simulink model "ModeAdjust"  (R2018b)
settings: Solver=FixedStepDiscrete  StartTime=0.0  StopTime=inf  FixedStep=0.01  RelTol=1e-3
undefined symbols (not defined in the file or in its folder): IfKeSMSbSeatMovBkRclnEnable_Val, IfKeSMSbSeatMovFrwdBkwdEnable_Val, IfKeSMSbSeatMovFtrstEnable_Val, IfKeSMSbSeatMovHdrstFrwdBkwdEnable_Val, IfKeSMSbSeatMovHdUpwdDnwdEnable_Val, IfKeSMSbSeatMovLgrstEnable_Val, IfKeSMSbSeatMovLtwdRtwdEnable_Val, IfVeSMSeStNumConfig, KeSMSbArmscreenMovEnable_Val, KeSMSbSeatMovLgrstExpdEnable_Val, KeSMSuFirstRwStBackPosDelta_Val, KeSMSuFirstRwStBackPosTolr_Val, KeSMSuFirstRwStCushFrntPosDelta_Val, KeSMSuFirstRwStCushFrntPosTolr_Val, KeSMSuFirstRwStCushRePosDelta_Val, KeSMSuFirstRwStCushRePosTolr_Val, KeSMSuFirstRwStFootrestPosDelta_Val, KeSMSuFirstRwStFootrestPosTolr_Val, KeSMSuFirstRwStFwdBkwdPosDelta_Val, KeSMSuFirstRwStFwdBkwdPosTolr_Val, KeSMSuMdMotFinshdTm_Val, KeSMSuMdRetryTm1_Val, KeSMSuModeReqDurgTm_Val, KeSMSuSecRwStArmTochPosDelta_Val, KeSMSuSecRwStArmTochPosTolr_Val, KeSMSuSecRwStBackPosDelta_Val, KeSMSuSecRwStBackPosTolr_Val, KeSMSuSecRwStFtrstUpwdDnwdPosDelta_Val, KeSMSuSecRwStFtrstUpwdDnwdPosTolr_Val, KeSMSuSecRwStFwdBkwdPosDelta_Val, KeSMSuSecRwStFwdBkwdPosTolr_Val, KeSMSuSecRwStHeadrestFwdBkwdPosDelta_Val, KeSMSuSecRwStHeadrestFwdBkwdPosTolr_Val, KeSMSuSecRwStHeadrestUpwdDwnwdPosDelta_Val, KeSMSuSecRwStHeadrestUpwdDwnwdPosTolr_Val, KeSMSuSecRwStLegrestInOutPosDelta_Val, KeSMSuSecRwStLegrestInOutPosTolr_Val, KeSMSuSecRwStLegrestUpwdDwnwdPosDelta_Val, KeSMSuSecRwStLegrestUpwdDwnwdPosTolr_Val, KeSMSuSecRwStLwdRwdPosDelta_Val, KeSMSuSecRwStLwdRwdPosTolr_Val, KeSMSuSecRwStVIPFtrstRefAngle_Val, KeSMSuThirdRwStFwdBkwdPosDelta_Val, KeSMSuThirdRwStFwdBkwdPosTolr_Val, KeSMSuThrdRwCushFoldPosDelta_Val, KeSMSuThrdRwCushFoldPosTolr_Val, KeSMSuThrdRwStBackPosDelta_Val, KeSMSuThrdRwStBackPosTolr_Val, KeSMSw4SLegrstCloseMdSecRwLtStFtrstUpwdDnwdPos_Val, KeSMSw4SLegrstCloseMdSecRwLtStFtrstUpwdDnwdPosMax_Val, KeSMSw4SLegrstCloseMdSecRwLtStFtrstUpwdDnwdPosMin_Val, KeSMSw4SLegrstCloseMdSecRwLtStLgrstOtwdInwdPos_Val, KeSMSw4SLegrstCloseMdSecRwLtStLgrstOtwdInwdPosMax_Val, KeSMSw4SLegrstCloseMdSecRwLtStLgrstOtwdInwdPosMin_Val, KeSMSw4SLegrstCloseMdSecRwLtStLgrstUpwdDnwdPos_Val, KeSMSw4SLegrstCloseMdSecRwLtStLgrstUpwdDnwdPosMax_Val, KeSMSw4SLegrstCloseMdSecRwLtStLgrstUpwdDnwdPosMin_Val, KeSMSw4SLegrstCloseMdSecRwRtStFtrstUpwdDnwdPos_Val, KeSMSw4SLegrstCloseMdSecRwRtStFtrstUpwdDnwdPosMax_Val, KeSMSw4SLegrstCloseMdSecRwRtStFtrstUpwdDnwdPosMin_Val ... (+1138)
libraries: Lib x401
(part 23 of 35)

== system ModeAdjust/ModeAdjustRunnable_sys/ModeAdjust/VIPR/R2Rt ==
  note: %1锁，2未锁
  Mode_Trig : Inport
  Step1En : Inport  Port=2
  Step2En : Inport  Port=3
  Step3En : Inport  Port=4
  SecRwRtStPoss : Inport  Port=5
  SecRwRtStPossV : Inport  Port=6
  SecRwRtStChldLkRsp_L : Inport  Port=7
  ModeStCalib_2R : Inport  Port=8
  StConfig : Inport  Port=9
  isSeatOccupied : Inport  Port=10
  Bus Creator : BusCreator  Inputs=9  OutDataTypeStr=Bus: SecRwRtSeatPos
  Bus Selector : BusSelector  OutputSignals=IfVeSMSuSecRwRtStBkReclnUpwdDnwdPos_Val_read,IfVeSMSuSecRwRtStFrwdBkwdPos_Val_read,IfVeSMSuSecRwRtStHPassStUpwdDnwdPos_Val_read,IfVeSMSuSecRwRtStLgrstUpwdDnwdPos_Val_read,IfVeSMSuSecRwRtStLtwdRtwdPos_Val_read,SecRwRtStArmScrnPos_Val_read
  Bus Selector1 : BusSelector  OutputSignals=IfVeSMSuSecRwRtStBkReclnUpwdDnwdPosV_Val_read,IfVeSMSuSecRwRtStFrwdBkwdPosV_Val_read,IfVeSMSuSecRwRtStHPassStUpwdDnwdPosV_Val_read,IfVeSMSuSecRwRtStLgrstUpwdDnwdPosV_Val_read,IfVeSMSuSecRwRtStLtwdRtwdPosV_Val_read,SecRwRtStArmScrnPosV_Val_read
  Bus Selector2 : BusSelector  OutputSignals=ArmScrnPos,ArmScrnPosMax,ArmScrnPosMin,BkReclnUpwdDnwdPos,BkReclnUpwdDnwdPosMax,BkReclnUpwdDnwdPosMin,FrwdBkwdPos,FrwdBkwdPosMax,FrwdBkwdPosMin,HdrstUpwdPos,HdrstUpwdPosMax,HdrstUpwdPosMin,LgrstUpwdPos,LgrstUpwdPosMax,LgrstUpwdPosMin,LtwdRtwdPos,LtwdRtwdPosMax,LtwdRtwdPosMin
  Bus Selector3 : BusSelector  OutputSignals=VIPSecRwRtSt
  Bus Selector4 : BusSelector  OutputSignals=BkReclnUpwdDnwdMovConfig,ArmTouchMovConfig,FrwdBkwdMovConfig,LgrstUpwdMovConfig,LtwdRtwdMovConfig
  Constant : Constant  Value=2  OutDataTypeStr=uint8
  Constant1 : Constant  Value=0  OutDataTypeStr=uint8
  Delay1 : Delay  DelayLength=1
  Delay2 : Delay  DelayLength=1
  Delay4 : Delay  DelayLength=1
  Logical Operator{1..3,5..6,10} (6 alike) : Logic  AllPortsSameDT=off  OutDataTypeStr=boolean
  Logical Operator{4,11..12,16} (4 alike) : Logic  Operator=OR  AllPortsSameDT=off  OutDataTypeStr=boolean
  Logical Operator15 : Logic  Inputs=3  AllPortsSameDT=off  OutDataTypeStr=boolean
  PA_KeSMSuMdMotFinshdTm_Val : Constant  Value=KeSMSuMdMotFinshdTm_Val
  PA_KeSMSuMdRetryTm1_Val : Constant  Value=KeSMSuMdRetryTm1_Val
  PA_KeSMSuModeReqDurgTm_Val : Constant  Value=KeSMSuModeReqDurgTm_Val
  PA_KeSMSuSecRwStArmTochPosDelta_Val : Constant  Value=KeSMSuSecRwStArmTochPosDelta_Val
  PA_KeSMSuSecRwStBackPosDelta_Val : Constant  Value=KeSMSuSecRwStBackPosDelta_Val
  PA_KeSMSuSecRwStFwdBkwdPosDelta_Val : Constant  Value=KeSMSuSecRwStFwdBkwdPosDelta_Val
  PA_KeSMSuSecRwStLegrestUpwdDwnwdPosDelta_Val : Constant  Value=KeSMSuSecRwStLegrestUpwdDwnwdPosDelta_Val
  PA_KeSMSuSecRwStLwdRwdPosDelta_Val : Constant  Value=KeSMSuSecRwStLwdRwdPosDelta_Val
  PA_KeSMSwDltTrgtPos_Val{1,3,6,10,12,17,19..22} (10 alike) : Constant  Value=KeSMSwPosInvalidVal_Val
  PA_KeSMSwDltTrgtPos_Val18 : Constant  OutDataTypeStr=boolean
  PA_KeSMSwDltTrgtPos_Val2 : Constant  Value=SeatChldLkSt.ChldLkSt_Unlock
  PA_KeSMSwDltTrgtPos_Val4 : Constant  Value=0  OutDataTypeStr=boolean
  PA_KeSMSwDltTrgtPos_Val5 : Constant  Value=0  OutDataTypeStr=boolean
  PA_KeSMSwDltTrgtPos_Val8 : Constant  Value=0  OutDataTypeStr=boolean
  R2LtSt_BkReclnUpwdDnwd_Lt_Step1 : Subsystem
  R2RtSt_LgrstUpwd_Step3 : Lib/CommonUsed  SystemSampleTime=-1
  R2Rt_LtwdRtwd_Step2 : Lib/CommonUsed  SystemSampleTime=-1
  Relational Operator : RelationalOperator  Operator=~=  OutDataTypeStr=boolean  RndMeth=Simplest
  Relational Operator2 : RelationalOperator  Operator=~=  OutDataTypeStr=boolean  RndMeth=Simplest
  SecRwRtStFrwdBkwd_Step2 : Lib/CommonUsed  SystemSampleTime=-1
  Switch : Switch  Criteria=u2 ~= 0
  Unit Delay : UnitDelay  SampleTime=-1
  R2RtSt_Step1_ini : Outport
  ini_ReclnOverUp : Outport  Port=2
  ini_ReclnOverDwn : Outport  Port=3
  R2RtSt_Step2_ini : Outport  Port=4
  R2Rt_Step1_done : Outport  Port=5
  R2Rt_Step2_done : Outport  Port=6
  R2Rt_TrgtPoss : Outport  Port=7  VectorParamsAs1DForOutWhenUnconnected=on
  R2RtSt_Step3_ini : Outport  Port=8
  R2Rt_Step3_done : Outport  Port=9
  IfVeSMSbSecRwRtStRclCmdSrv_Val_writeRaw : Outport  Port=10
  R2Rt_All_done : Outport  Port=11
  R2Rt_SpdCtrl : Outport  Port=12  VectorParamsAs1DForOutWhenUnconnected=on
  wires:
  PA_KeSMSwDltTrgtPos_Val8/1 -> R2Rt_LtwdRtwd_Step2/13
  PA_KeSMSwDltTrgtPos_Val5/1 -> SecRwRtStFrwdBkwd_Step2/13
  PA_KeSMSwDltTrgtPos_Val4/1 -> R2RtSt_LgrstUpwd_Step3/13
  ModeStCalib_2R/1 -> Bus Selector3/1
  Bus Selector2/6 -> [K_BkReclnUpwdDnwdPosMin]  "<BkReclnUpwdDnwdPosMin>"
  Bus Selector2/2 -> [K_ArmScrnPosMax]  "<ArmScrnPosMax>"
  Bus Selector2/3 -> [K_ArmScrnPosMin]  "<ArmScrnPosMin>"
  Bus Selector2/7 -> [K_FrwdBkwdPos]  "<FrwdBkwdPos>"
  Bus Selector3/1 -> Bus Selector2/1  "<VIPSecRwRtSt>"
  Bus Selector2/8 -> [K_FrwdBkwdPosMax]  "<FrwdBkwdPosMax>"
  Bus Selector2/5 -> [K_BkReclnUpwdDnwdPosMax]  "<BkReclnUpwdDnwdPosMax>"
  Bus Selector2/9 -> [K_FrwdBkwdPosMin]  "<FrwdBkwdPosMin>"
  Bus Selector2/4 -> [K_BkReclnUpwdDnwdPos]  "<BkReclnUpwdDnwdPos>"
  Bus Selector2/10 -> [K_HdrstUpwdPos]  "<HdrstUpwdPos>"
  Bus Selector2/14 -> [K_LgrstUpwdPosMax]  "<LgrstUpwdPosMax>"
  Bus Selector2/11 -> [K_HdrstUpwdPosMax]  "<HdrstUpwdPosMax>"
  Bus Selector2/13 -> [K_LgrstUpwdPos]  "<LgrstUpwdPos>"
  Bus Selector2/12 -> [K_HdrstUpwdPosMin]  "<HdrstUpwdPosMin>"
  Bus Selector2/17 -> [K_LtwdRtwdPosMax]  "<LtwdRtwdPosMax>"
  Bus Selector2/15 -> [K_LgrstUpwdPosMin]  "<LgrstUpwdPosMin>"
  Bus Selector2/16 -> [K_LtwdRtwdPos]  "<LtwdRtwdPos>"
  Bus Selector2/18 -> [K_LtwdRtwdPosMin]  "<LtwdRtwdPosMin>"
  Bus Selector2/1 -> [K_ArmScrnPos]  "<ArmScrnPos>"
  Bus Selector1/6 -> [SecRwRtStArmScrnPosV]  "<SecRwRtStArmScrnPosV_Val_read>"
  Bus Selector/6 -> [SecRwRtStArmScrnPos]  "<SecRwRtStArmScrnPos_Val_read>"
  [KeSMSuMdMotFinshdTm_Val] -> SecRwRtStFrwdBkwd_Step2/12
  [KeSMSuMdMotFinshdTm_Val] -> R2Rt_LtwdRtwd_Step2/12
  [KeSMSuMdMotFinshdTm_Val] -> R2RtSt_LgrstUpwd_Step3/12
  [KeSMSuMdMotFinshdTm_Val] -> R2LtSt_BkReclnUpwdDnwd_Lt_Step1/13(CheckFinishTm)
  PA_KeSMSuSecRwStArmTochPosDelta_Val/1 -> [KeSMSuSecRwStArmTochPosDelta_Val]
  PA_KeSMSuMdMotFinshdTm_Val/1 -> [KeSMSuMdMotFinshdTm_Val]
  PA_KeSMSuSecRwStBackPosDelta_Val/1 -> [KeSMSuSecRwStBackPosDelta_Val]
  PA_KeSMSuSecRwStLwdRwdPosDelta_Val/1 -> [KeSMSuSecRwStLwdRwdPosDelta_Val]
  PA_KeSMSuSecRwStLegrestUpwdDwnwdPosDelta_Val/1 -> [KeSMSuSecRwStLegrestUpwdDwnwdPosDelta_Val]
  PA_KeSMSuSecRwStFwdBkwdPosDelta_Val/1 -> [KeSMSuSecRwStFwdBkwdPosDelta_Val]
  PA_KeSMSwDltTrgtPos_Val1/1 -> Bus Creator/9  "SecRwRtStArmScrnTrgtPos"
  [Step3_1_done] -> Logical Operator10/1
  R2LtSt_BkReclnUpwdDnwd_Lt_Step1/7(Stg_done3) -> [Step3_1_done]
  R2LtSt_BkReclnUpwdDnwd_Lt_Step1/5(TarPos) -> [R2RtSt_BkReclnUpwdDnwd_TarPos]
  [Step3En] -> R2LtSt_BkReclnUpwdDnwd_Lt_Step1/3(Ena3)
  [Step1En] -> R2LtSt_BkReclnUpwdDnwd_Lt_Step1/2(Ena1)
  PA_KeSMSuModeReqDurgTm_Val/1 -> [Tick]
  [SecRwRtStLtwdRtwdPosV] -> R2Rt_LtwdRtwd_Step2/8
  [K_LgrstUpwdPos] -> R2RtSt_LgrstUpwd_Step3/6
  [K_LgrstUpwdPosMax] -> R2RtSt_LgrstUpwd_Step3/5
  [K_LgrstUpwdPosMin] -> R2RtSt_LgrstUpwd_Step3/4
  [Step3done] -> Logical Operator15/3
  [Step2done] -> Logical Operator15/2
  [Step1done_1] -> Logical Operator15/1
  [R2Rt_Step3_2_ini] -> Logical Operator16/1
  Unit Delay/1 -> Logical Operator16/2
  Logical Operator15/1 -> R2Rt_All_done/1
  Logical Operator12/1 -> R2Rt_Step3_done/1, [Step3done]
  PA_KeSMSwDltTrgtPos_Val18/1 -> IfVeSMSbSecRwRtStRclCmdSrv_Val_writeRaw/1
  [R2RtSt_Step3_ini] -> Logical Operator12/1
  [R2RtSt_Step2_ini] -> Logical Operator11/1
  Delay1/1 -> Logical Operator11/2
  Logical Operator11/1 -> R2Rt_Step2_done/1, [Step2done]
  [Step3_2_done] -> Logical Operator10/2
  Logical Operator10/1 -> Logical Operator2/2
  [Step2done] -> Delay4/1
  Delay2/1 -> Logical Operator12/2
  Logical Operator3/1 -> Logical Operator5/2
  Logical Operator5/1 -> Delay1/1
  [Step1done_1] -> Logical Operator5/1
  Logical Operator16/1 -> R2Rt_Step1_done/1, [Step1done_1]
  [Step2En] -> SecRwRtStFrwdBkwd_Step2/2
  [Step3En] -> R2RtSt_LgrstUpwd_Step3/2
  Step3En/1 -> [Step3En]
  Logical Operator2/1 -> Delay2/1
  [R2Rt_Step3_2_ini] -> Logical Operator1/2
  [R2Rt_Step3_1_ini] -> Logical Operator1/1
  R2RtSt_LgrstUpwd_Step3/1 -> [R2Rt_Step3_1_ini]
  Logical Operator1/1 -> R2RtSt_Step3_ini/1, [R2RtSt_Step3_ini]
  R2LtSt_BkReclnUpwdDnwd_Lt_Step1/3(ini_ReclnOverDwn) -> ini_ReclnOverDwn/1
  R2LtSt_BkReclnUpwdDnwd_Lt_Step1/2(ini_ReclnOverUp) -> ini_ReclnOverUp/1
  R2LtSt_BkReclnUpwdDnwd_Lt_Step1/1(ini_st) -> R2RtSt_Step1_ini/1, [R2Rt_Step3_2_ini]
  R2RtSt_LgrstUpwd_Step3/4 -> [Step3_2_done]
  R2RtSt_LgrstUpwd_Step3/3 -> [R2RtSt_LgrstUpwd_TarPos]
  R2RtSt_LgrstUpwd_Step3/2 -> [Step1_2_ArrivedTarPos]
  [Tick] -> R2RtSt_LgrstUpwd_Step3/11
  PA_KeSMSwDltTrgtPos_Val12/1 -> R2RtSt_LgrstUpwd_Step3/10
  [SecRwRtStLgrstUpwdDnwdPosV] -> R2RtSt_LgrstUpwd_Step3/8
  [KeSMSuSecRwStLegrestUpwdDwnwdPosDelta_Val] -> R2RtSt_LgrstUpwd_Step3/7
  [SecRwRtStBkReclnUpwdDnwdPosV] -> R2LtSt_BkReclnUpwdDnwd_Lt_Step1/9(PosValid)
  [SecRwRtStLgrstUpwdDnwdPos] -> R2RtSt_LgrstUpwd_Step3/3
  [Trig] -> R2RtSt_LgrstUpwd_Step3/1
  PA_KeSMSwDltTrgtPos_Val2/1 -> Relational Operator/2
  SecRwRtStChldLkRsp_L/1 -> Relational Operator/1
  SecRwRtStFrwdBkwd_Step2/4 -> [Step2done_1]
  [Tick] -> SecRwRtStFrwdBkwd_Step2/11
  [Tick] -> R2LtSt_BkReclnUpwdDnwd_Lt_Step1/12(Tick)
  PA_KeSMSwDltTrgtPos_Val6/1 -> SecRwRtStFrwdBkwd_Step2/10
  [ChildLocker] -> SecRwRtStFrwdBkwd_Step2/9
  [ChildLocker] -> R2LtSt_BkReclnUpwdDnwd_Lt_Step1/10(ChildLocker)
  [SecRwRtStFrwdBkwdPosV] -> SecRwRtStFrwdBkwd_Step2/8
  [K_FrwdBkwdPos] -> SecRwRtStFrwdBkwd_Step2/6
  [Trig] -> SecRwRtStFrwdBkwd_Step2/1
  PA_KeSMSwDltTrgtPos_Val3/1 -> R2LtSt_BkReclnUpwdDnwd_Lt_Step1/11(InvalidValue)
  [K_BkReclnUpwdDnwdPos] -> R2LtSt_BkReclnUpwdDnwd_Lt_Step1/7(Tar_Pos)
  [SecRwRtStBkReclnUpwdDnwdPos] -> R2LtSt_BkReclnUpwdDnwd_Lt_Step1/4(Current_Pos)
  R2LtSt_BkReclnUpwdDnwd_Lt_Step1/4(isArrivedTarPos) -> [Step1_3_ArrivedTarPos], [Step1_1_ArrivedTarPos]
  [K_BkReclnUpwdDnwdPosMin] -> R2LtSt_BkReclnUpwdDnwd_Lt_Step1/5(Calib_Min)
  SecRwRtStFrwdBkwd_Step2/2 -> [Step2_1_ArrivedTarPos]
  SecRwRtStFrwdBkwd_Step2/1 -> [FrwdBkwd_inidone_Step2]
  [K_FrwdBkwdPosMin] -> SecRwRtStFrwdBkwd_Step2/4
  [KeSMSuSecRwStFwdBkwdPosDelta_Val] -> SecRwRtStFrwdBkwd_Step2/7
  [K_FrwdBkwdPosMax] -> SecRwRtStFrwdBkwd_Step2/5
  [SecRwRtStFrwdBkwdPos] -> SecRwRtStFrwdBkwd_Step2/3
  [KeSMSuSecRwStBackPosDelta_Val] -> R2LtSt_BkReclnUpwdDnwd_Lt_Step1/8(Tar_PosDelta)
  Mode_Trig/1 -> [Trig]
  [Trig] -> R2LtSt_BkReclnUpwdDnwd_Lt_Step1/1(MSM_Trig)
  [K_BkReclnUpwdDnwdPosMax] -> R2LtSt_BkReclnUpwdDnwd_Lt_Step1/6(Calib_Max)
  Bus Selector1/2 -> [SecRwRtStFrwdBkwdPosV]  "<IfVeSMSuSecRwRtStFrwdBkwdPosV_Val_read>"
  SecRwRtStPossV/1 -> Bus Selector1/1
  Bus Selector1/3 -> [SecRwRtStHPassStUpwdDnwdPosV]  "<IfVeSMSuSecRwRtStHPassStUpwdDnwdPosV_Val_read>"
  Bus Selector/4 -> [SecRwRtStLgrstUpwdDnwdPos]  "<IfVeSMSuSecRwRtStLgrstUpwdDnwdPos_Val_read>"
  Bus Selector1/1 -> [SecRwRtStBkReclnUpwdDnwdPosV]  "<IfVeSMSuSecRwRtStBkReclnUpwdDnwdPosV_Val_read>"
  Bus Selector/1 -> [SecRwRtStBkReclnUpwdDnwdPos]  "<IfVeSMSuSecRwRtStBkReclnUpwdDnwdPos_Val_read>"
  Bus Selector1/4 -> [SecRwRtStLgrstUpwdDnwdPosV]  "<IfVeSMSuSecRwRtStLgrstUpwdDnwdPosV_Val_read>"
  Bus Selector/5 -> [SecRwRtStLtwdRtwdPos]  "<IfVeSMSuSecRwRtStLtwdRtwdPos_Val_read>"
  SecRwRtStPoss/1 -> Bus Selector/1
  Bus Selector1/5 -> [SecRwRtStLtwdRtwdPosV]  "<IfVeSMSuSecRwRtStLtwdRtwdPosV_Val_read>"
  Bus Selector/3 -> [SecRwRtStHPassStUpwdDnwdPos]  "<IfVeSMSuSecRwRtStHPassStUpwdDnwdPos_Val_read>"
  Bus Selector/2 -> [SecRwRtStFrwdBkwdPos]  "<IfVeSMSuSecRwRtStFrwdBkwdPos_Val_read>"
  SecRwRtStFrwdBkwd_Step2/3 -> [R2Rt_StFrwdBkwd_TarPos]
  [Trig] -> R2Rt_LtwdRtwd_Step2/1
  [Step2En] -> R2Rt_LtwdRtwd_Step2/2
  [SecRwRtStLtwdRtwdPos] -> R2Rt_LtwdRtwd_Step2/3
  [K_LtwdRtwdPosMin] -> R2Rt_LtwdRtwd_Step2/4
  [K_LtwdRtwdPosMax] -> R2Rt_LtwdRtwd_Step2/5
  [K_LtwdRtwdPos] -> R2Rt_LtwdRtwd_Step2/6
  [KeSMSuSecRwStLwdRwdPosDelta_Val] -> R2Rt_LtwdRtwd_Step2/7
  [ChildLocker] -> R2Rt_LtwdRtwd_Step2/9
  PA_KeSMSwDltTrgtPos_Val17/1 -> R2Rt_LtwdRtwd_Step2/10
  [Tick] -> R2Rt_LtwdRtwd_Step2/11
  R2Rt_LtwdRtwd_Step2/3 -> [R2Rt_LtwdRtwd_TarPos]
  R2Rt_LtwdRtwd_Step2/1 -> [LtwdRtwd_inidone_Step2]
  R2Rt_LtwdRtwd_Step2/2 -> [Step2_2_ArrivedTarPos]
  R2Rt_LtwdRtwd_Step2/4 -> [Step2done_2]
  [FrwdBkwd_inidone_Step2] -> Logical Operator6/1
  [LtwdRtwd_inidone_Step2] -> Logical Operator6/2
  Logical Operator6/1 -> R2RtSt_Step2_ini/1, [R2RtSt_Step2_ini]
  R2LtSt_BkReclnUpwdDnwd_Lt_Step1/6(Stg_done1) -> Unit Delay/1
  [Step2done_1] -> Logical Operator3/1
  [Step2done_2] -> Logical Operator3/2
  Bus Creator/1 -> R2Rt_TrgtPoss/1
  [R2Rt_StFrwdBkwd_TarPos] -> Bus Creator/5  "SecRwRtStFrwdBkwdTrgtPos"
  [R2Rt_LtwdRtwd_TarPos] -> Bus Creator/8  "SecRwRtStLtwdRtwdTrgtPos"
  PA_KeSMSwDltTrgtPos_Val22/1 -> Bus Creator/6  "SecRwRtStHdrstUpwdDnwdTrgtPos"
  [R2RtSt_LgrstUpwd_TarPos] -> Bus Creator/7  "SecRwRtStLgrstUpwdDnwdTrgtPos"
  PA_KeSMSwDltTrgtPos_Val19/1 -> Bus Creator/2  "SecRwRtStBlstOtwdInwdTrgtPos"
  [R2RtSt_BkReclnUpwdDnwd_TarPos] -> Bus Creator/1  "SecRwRtStBkReclnUpwdDnwdTrgtPos"
  PA_KeSMSwDltTrgtPos_Val20/1 -> Bus Creator/3  "SecRwRtStCshnFrntUpwdDnwdTrgtPos"
  PA_KeSMSwDltTrgtPos_Val21/1 -> Bus Creator/4  "SecRwRtStCshnRrUpwdDnwdTrgtPos"
  Step1En/1 -> [Step1En]
  Step2En/1 -> [Step2En]
  Delay4/1 -> Logical Operator2/1
  StConfig/1 -> Bus Selector4/1
  Bus Selector4/3 -> [FrwdBkwdMovConfig]  "<FrwdBkwdMovConfig>"
  Bus Selector4/5 -> [LtwdRtwdMovConfig]  "<LtwdRtwdMovConfig>"
  Bus Selector4/4 -> [LgrstUpwdMovConfig]  "<LgrstUpwdMovConfig>"
  Bus Selector4/2 -> [ArmTouchMovConfig]  "<ArmTouchMovConfig>"
  Bus Selector4/1 -> [BkReclnUpwdDnwdMovConfig]  "<BkReclnUpwdDnwdMovConfig>"
  [LtwdRtwdMovConfig] -> R2Rt_LtwdRtwd_Step2/14
  [FrwdBkwdMovConfig] -> SecRwRtStFrwdBkwd_Step2/14
  [LgrstUpwdMovConfig] -> R2RtSt_LgrstUpwd_Step3/14
  [BkReclnUpwdDnwdMovConfig] -> R2LtSt_BkReclnUpwdDnwd_Lt_Step1/14(StConfig)
  [ChildLocker] -> R2RtSt_LgrstUpwd_Step3/9
  Relational Operator/1 -> Logical Operator4/2
  isSeatOccupied/1 -> Logical Operator4/1
  Logical Operator4/1 -> [ChildLocker]
  [CntLow] -> R2RtSt_LgrstUpwd_Step3/15
  [CntLow] -> R2Rt_LtwdRtwd_Step2/15
  [CntLow] -> SecRwRtStFrwdBkwd_Step2/15
  PA_KeSMSuMdRetryTm1_Val/1 -> [CntLow]
  Relational Operator2/1 -> Switch/2
  [R2Rt_StFrwdBkwd_TarPos] -> Relational Operator2/1
  Constant1/1 -> Switch/3
  Constant/1 -> Switch/1
  PA_KeSMSwDltTrgtPos_Val10/1 -> Relational Operator2/2
  Switch/1 -> R2Rt_SpdCtrl/1

== system ModeAdjust/ModeAdjustRunnable_sys/ModeAdjust/VIPR/R3Lt ==
  note: %1锁，2未锁
  Mode_Trig : Inport
  Step1En : Inport  Port=2
  isSeatOccupied : Inport  Port=3
  ThdRwLtStPoss : Inport  Port=4
  ThdRwLtStPossV : Inport  Port=5
  ModeStCalib_3L : Inport  Port=6
  is6s : Inport  Port=7
  StConfig : Inport  Port=8
  SecRwRtStChldLkRsp_L : Inport  Port=9
  Bus Creator : BusCreator  Inputs=3  OutDataTypeStr=Bus: ThdRwLfSeatPos
  Bus Selector : BusSelector  OutputSignals=IfVeSMSuThdRwLtStBkReclnUpwdDnwdPos_Val_read,IfVeSMSuThdRwLtStCshnFldUpwdDnwdPos_Val_read,IfVeSMSuThdRwLtStFrwdBkwdPos_Val_read
  Bus Selector1 : BusSelector  OutputSignals=IfVeSMSuThdRwLtStBkReclnUpwdDnwdPosV_Val_read,IfVeSMSuThdRwLtStCshnFldUpwdDnwdPosV_Val_read,IfVeSMSuThdRwLtStFrwdBkwdPosV_Val_read
  Bus Selector2 : BusSelector  OutputSignals=BkReclnUpwdDnwdPos,BkReclnUpwdDnwdPosMax,BkReclnUpwdDnwdPosMin,CshnFldUpwdDnwdPos,CshnFldUpwdDnwdPosMax,CshnFldUpwdDnwdPosMin,FrwdBkwdPos,FrwdBkwdPosMax,FrwdBkwdPosMin
  Bus Selector3 : BusSelector  OutputSignals=VIPThdRwLtSt
  Bus Selector4 : BusSelector  OutputSignals=BkReclnUpwdDnwdMovConfig,CshnFldUpwdDnwdMovConfig,FrwdBkwdMovConfig
  Constant : Constant  Value=3  OutDataTypeStr=uint8
  Constant1 : Constant  Value=2  OutDataTypeStr=uint8
  Delay2 : Delay  DelayLength=1
  Logical Operator : Logic  AllPortsSameDT=off  OutDataTypeStr=boolean
  Logical Operator4 : Logic  AllPortsSameDT=off  OutDataTypeStr=boolean
  Logical Operator6 : Logic  Operator=OR  AllPortsSameDT=off  OutDataTypeStr=boolean
  Logical Operator8 : Logic  Operator=OR  AllPortsSameDT=off  OutDataTypeStr=boolean
  PA_KeSMSuMdMotFinshdTm_Val : Constant  Value=KeSMSuMdMotFinshdTm_Val
  PA_KeSMSuMdRetryTm1_Val : Constant  Value=KeSMSuMdRetryTm1_Val
  PA_KeSMSuModeReqDurgTm_Val : Constant  Value=KeSMSuModeReqDurgTm_Val
  PA_KeSMSuThirdRwStFwdBkwdPosDelta_Val : Constant  Value=KeSMSuThirdRwStFwdBkwdPosDelta_Val
  PA_KeSMSuThrdRwCushFoldPosDelta_Val : Constant  Value=KeSMSuThrdRwCushFoldPosDelta_Val
  PA_KeSMSuThrdRwStBackPosDelta_Val : Constant  Value=KeSMSuThrdRwStBackPosDelta_Val
  PA_KeSMSwDltTrgtPos_Val11 : Constant  Value=SeatChldLkSt.ChldLkSt_Unlock
  PA_KeSMSwDltTrgtPos_Val13 : Constant  Value=0  OutDataTypeStr=boolean
  PA_KeSMSwDltTrgtPos_Val{3,6,8,18} (4 alike) : Constant  Value=KeSMSwPosInvalidVal_Val
  PA_KeSMSwDltTrgtPos_Val4 : Constant  OutDataTypeStr=boolean
  R3LtSt_BkReclnUpwdDnwd_Step1 : Lib/CommonUsed  SystemSampleTime=-1
  R3Lt_FrwdBkwd_Step1 : Lib/CommonUsed  SystemSampleTime=-1
  Relational Operator1 : RelationalOperator  Operator=~=  OutDataTypeStr=boolean  RndMeth=Simplest
  Relational Operator5 : RelationalOperator  Operator=~=  OutDataTypeStr=boolean  RndMeth=Simplest
  Switch : Switch  Criteria=u2 > Threshold
  Switch1 : Switch  Criteria=u2 ~= 0
  R3Lt_Step1_ini : Outport
  R3Lt_Step1done : Outport  Port=2
  IfVeSMSbThdRwLtStRclCmdSrv_Val_writeRaw : Outport  Port=3
  R3Lt_TrgtPoss : Outport  Port=4  VectorParamsAs1DForOutWhenUnconnected=on
  R3Lt_All_done : Outport  Port=5
  R3Lt_SpdCtrl : Outport  Port=6  VectorParamsAs1DForOutWhenUnconnected=on
  wires:
  Bus Creator/1 -> R3Lt_TrgtPoss/1
  [R3Lt_BkReclnUpwdDnwd_TarPos] -> Bus Creator/1  "ThdRwLtStBkReclnUpwdDnwdTrgtPos"
  PA_KeSMSwDltTrgtPos_Val8/1 -> Bus Creator/2  "ThdRwLtStCshnFldUpwdDnwdTrgtPos"
  [R3LtFrwdBkwd_TarPos] -> Bus Creator/3  "ThdRwLtStFrwdBkwdTrgtPos"
  Bus Selector/1 -> [ThdRwLtStBkReclnUpwdDnwdPos]  "<IfVeSMSuThdRwLtStBkReclnUpwdDnwdPos_Val_read>"
  Bus Selector1/1 -> [ThdRwLtStBkReclnUpwdDnwdPosV]  "<IfVeSMSuThdRwLtStBkReclnUpwdDnwdPosV_Val_read>"
  ThdRwLtStPossV/1 -> Bus Selector1/1
  Bus Selector1/3 -> [ThdRwLtStFrwdBkwdPosV]  "<IfVeSMSuThdRwLtStFrwdBkwdPosV_Val_read>"
  Bus Selector/3 -> [ThdRwLtStFrwdBkwdPos]  "<IfVeSMSuThdRwLtStFrwdBkwdPos_Val_read>"
  ThdRwLtStPoss/1 -> Bus Selector/1
  Bus Selector1/2 -> [ThdRwLtStCshnFldUpwdDnwdPosV]  "<IfVeSMSuThdRwLtStCshnFldUpwdDnwdPosV_Val_read>"
  Bus Selector/2 -> [ThdRwLtStCshnFldUpwdDnwdPos]  "<IfVeSMSuThdRwLtStCshnFldUpwdDnwdPos_Val_read>"
  [K_BkReclnUpwdDnwdPosMax] -> R3LtSt_BkReclnUpwdDnwd_Step1/5
  [Trig] -> R3LtSt_BkReclnUpwdDnwd_Step1/1
  Mode_Trig/1 -> [Trig]
  [KeSMSuThrdRwStBackPosDelta_Val] -> R3LtSt_BkReclnUpwdDnwd_Step1/7
  [ThdRwLtStFrwdBkwdPos] -> R3Lt_FrwdBkwd_Step1/3
  [K_FrwdBkwdPosMax] -> R3Lt_FrwdBkwd_Step1/5
  [KeSMSuThirdRwStFwdBkwdPosDelta_Val] -> R3Lt_FrwdBkwd_Step1/7
  [K_FrwdBkwdPosMin] -> R3Lt_FrwdBkwd_Step1/4
  R3Lt_FrwdBkwd_Step1/1 -> [R3Lt_Step1_2_ini]
  R3Lt_FrwdBkwd_Step1/2 -> [Step2ArrivedTarPos]
  [K_BkReclnUpwdDnwdPosMin] -> R3LtSt_BkReclnUpwdDnwd_Step1/4
  R3LtSt_BkReclnUpwdDnwd_Step1/2 -> [Step1ArrivedTarPos]
  [ThdRwLtStBkReclnUpwdDnwdPos] -> R3LtSt_BkReclnUpwdDnwd_Step1/3
  [K_BkReclnUpwdDnwdPos] -> R3LtSt_BkReclnUpwdDnwd_Step1/6
  [ThdRwLtStBkReclnUpwdDnwdPosV] -> R3LtSt_BkReclnUpwdDnwd_Step1/8
  PA_KeSMSwDltTrgtPos_Val3/1 -> R3LtSt_BkReclnUpwdDnwd_Step1/10
  R3LtSt_BkReclnUpwdDnwd_Step1/3 -> [R3Lt_BkReclnUpwdDnwd_TarPos]
  R3LtSt_BkReclnUpwdDnwd_Step1/4 -> [Step1_1_done]
  Step1En/1 -> [Step1En], R3LtSt_BkReclnUpwdDnwd_Step1/2
  [Trig] -> R3Lt_FrwdBkwd_Step1/1
  [Step1En] -> R3Lt_FrwdBkwd_Step1/2
  [K_FrwdBkwdPos] -> R3Lt_FrwdBkwd_Step1/6
  [ThdRwLtStFrwdBkwdPosV] -> R3Lt_FrwdBkwd_Step1/8
  [isSeatOccupied] -> R3LtSt_BkReclnUpwdDnwd_Step1/9
  [isSeatOccupied] -> R3Lt_FrwdBkwd_Step1/9
  PA_KeSMSwDltTrgtPos_Val6/1 -> R3Lt_FrwdBkwd_Step1/10
  [Tick] -> R3LtSt_BkReclnUpwdDnwd_Step1/11
  [Tick] -> R3Lt_FrwdBkwd_Step1/11
  R3Lt_FrwdBkwd_Step1/3 -> [R3LtFrwdBkwd_TarPos]
  R3Lt_FrwdBkwd_Step1/4 -> [Step1_2_done]
  [Step1_2_done] -> Logical Operator4/2
  [Step1_1_done] -> Logical Operator4/1
  Logical Operator4/1 -> Delay2/1
  R3LtSt_BkReclnUpwdDnwd_Step1/1 -> [R3Lt_Step1_1_ini]
  [R3Lt_Step1_1_ini] -> Logical Operator/1
  [R3Lt_Step1_2_ini] -> Logical Operator/2
  Logical Operator/1 -> Logical Operator6/1, R3Lt_Step1_ini/1
  Logical Operator6/1 -> R3Lt_Step1done/1, [R3Lt_Step1_done]
  Delay2/1 -> Logical Operator6/2
  [R3Lt_Step1_done] -> R3Lt_All_done/1
  PA_KeSMSuModeReqDurgTm_Val/1 -> [Tick]
  PA_KeSMSuThrdRwCushFoldPosDelta_Val/1 -> [KeSMSuThrdRwCushFoldPosDelta_Val]
  PA_KeSMSuThirdRwStFwdBkwdPosDelta_Val/1 -> [KeSMSuThirdRwStFwdBkwdPosDelta_Val]
  PA_KeSMSuThrdRwStBackPosDelta_Val/1 -> [KeSMSuThrdRwStBackPosDelta_Val]
  PA_KeSMSuMdMotFinshdTm_Val/1 -> [KeSMSuMdMotFinshdTm_Val]
  [KeSMSuMdMotFinshdTm_Val] -> R3LtSt_BkReclnUpwdDnwd_Step1/12
  [KeSMSuMdMotFinshdTm_Val] -> R3Lt_FrwdBkwd_Step1/12
  Bus Selector2/6 -> [K_CshnFldUpwdDnwdPosMin]  "<CshnFldUpwdDnwdPosMin>"
  Bus Selector2/4 -> [K_CshnFldUpwdDnwdPos]  "<CshnFldUpwdDnwdPos>"
  Bus Selector2/7 -> [K_FrwdBkwdPos]  "<FrwdBkwdPos>"
  Bus Selector2/5 -> [K_CshnFldUpwdDnwdPosMax]  "<CshnFldUpwdDnwdPosMax>"
  ModeStCalib_3L/1 -> Bus Selector3/1
  Bus Selector2/3 -> [K_BkReclnUpwdDnwdPosMin]  "<BkReclnUpwdDnwdPosMin>"
  Bus Selector3/1 -> Bus Selector2/1  "<VIPThdRwLtSt>"
  Bus Selector2/9 -> [K_FrwdBkwdPosMin]  "<FrwdBkwdPosMin>"
  Bus Selector2/2 -> [K_BkReclnUpwdDnwdPosMax]  "<BkReclnUpwdDnwdPosMax>"
  Bus Selector2/1 -> [K_BkReclnUpwdDnwdPos]  "<BkReclnUpwdDnwdPos>"
  Bus Selector2/8 -> [K_FrwdBkwdPosMax]  "<FrwdBkwdPosMax>"
  is6s/1 -> [is6s]
  [is6s] -> R3Lt_FrwdBkwd_Step1/13
  [is6s] -> R3LtSt_BkReclnUpwdDnwd_Step1/13
  Bus Selector4/1 -> [BkReclnUpwdDnwdMovConfig]  "<BkReclnUpwdDnwdMovConfig>"
  StConfig/1 -> Bus Selector4/1
  Bus Selector4/2 -> [CshnFldUpwdDnwdMovConfig]  "<CshnFldUpwdDnwdMovConfig>"
  Bus Selector4/3 -> [FrwdBkwdMovConfig]  "<FrwdBkwdMovConfig>"
  [FrwdBkwdMovConfig] -> R3Lt_FrwdBkwd_Step1/14
  [BkReclnUpwdDnwdMovConfig] -> R3LtSt_BkReclnUpwdDnwd_Step1/14
  PA_KeSMSwDltTrgtPos_Val11/1 -> Relational Operator1/2
  SecRwRtStChldLkRsp_L/1 -> Relational Operator1/1
  Relational Operator1/1 -> Logical Operator8/1
  isSeatOccupied/1 -> Logical Operator8/2
  Logical Operator8/1 -> [isSeatOccupied]
  [is6s] -> Switch/2
  Switch/1 -> IfVeSMSbThdRwLtStRclCmdSrv_Val_writeRaw/1
  [CntLow] -> R3LtSt_BkReclnUpwdDnwd_Step1/15
  [CntLow] -> R3Lt_FrwdBkwd_Step1/15
  PA_KeSMSuMdRetryTm1_Val/1 -> [CntLow]
  Constant/1 -> Switch1/1
  Relational Operator5/1 -> Switch1/2
  PA_KeSMSwDltTrgtPos_Val18/1 -> Relational Operator5/2
  Constant1/1 -> Switch1/3
  [R3LtFrwdBkwd_TarPos] -> Relational Operator5/1  "ThdRwLtStFrwdBkwdTrgtPos"
  Switch1/1 -> R3Lt_SpdCtrl/1
  PA_KeSMSwDltTrgtPos_Val4/1 -> Switch/3
  PA_KeSMSwDltTrgtPos_Val13/1 -> Switch/1

== system ModeAdjust/ModeAdjustRunnable_sys/ModeAdjust/VIPR/R3Rt ==
  note: %1锁，2未锁
  Mode_Trig : Inport
  Step1En : Inport  Port=2
  SeatOccupied : Inport  Port=3
  ThdRwRtStPoss : Inport  Port=4
  ThdRwRtStPossV : Inport  Port=5
  ModeStCalib_3R : Inport  Port=6
  StConfig : Inport  Port=7
  SecRwRtStChldLkRsp_L : Inport  Port=8
  Bus Creator : BusCreator  Inputs=3  OutDataTypeStr=Bus: ThdRwRtSeatPos
  Bus Selector : BusSelector  OutputSignals=IfVeSMSuThdRwRtStBkReclnUpwdDnwdPos_Val_read,IfVeSMSuThdRwRtStCshnFldUpwdDnwdPos_Val_read,IfVeSMSuThdRwRtStFrwdBkwdPos_Val_read
  Bus Selector1 : BusSelector  OutputSignals=IfVeSMSuThdRwRtStBkReclnUpwdDnwdPosV_Val_read,IfVeSMSuThdRwRtStCshnFldUpwdDnwdPosV_Val_read,IfVeSMSuThdRwRtStFrwdBkwdPosV_Val_read
  Bus Selector2 : BusSelector  OutputSignals=BkReclnUpwdDnwdPos,BkReclnUpwdDnwdPosMax,BkReclnUpwdDnwdPosMin,CshnFldUpwdDnwdPos,CshnFldUpwdDnwdPosMax,CshnFldUpwdDnwdPosMin,FrwdBkwdPos,FrwdBkwdPosMax,FrwdBkwdPosMin
  Bus Selector3 : BusSelector  OutputSignals=VIPThdRwRtSt
  Bus Selector4 : BusSelector  OutputSignals=BkReclnUpwdDnwdMovConfig,CshnFldUpwdDnwdMovConfig,FrwdBkwdMovConfig
  Constant : Constant  Value=3  OutDataTypeStr=uint8
  Constant1 : Constant  Value=2  OutDataTypeStr=uint8
  Logical Operator : Logic  AllPortsSameDT=off  OutDataTypeStr=boolean
  Logical Operator4 : Logic  AllPortsSameDT=off  OutDataTypeStr=boolean
  Logical Operator6 : Logic  Operator=OR  AllPortsSameDT=off  OutDataTypeStr=boolean
  Logical Operator9 : Logic  Operator=OR  AllPortsSameDT=off  OutDataTypeStr=boolean
  PA_KeSMSuMdMotFinshdTm_Val : Constant  Value=KeSMSuMdMotFinshdTm_Val
  PA_KeSMSuMdRetryTm1_Val : Constant  Value=KeSMSuMdRetryTm1_Val
  PA_KeSMSuModeReqDurgTm_Val : Constant  Value=KeSMSuModeReqDurgTm_Val
  PA_KeSMSuThirdRwStFwdBkwdPosDelta_Val : Constant  Value=KeSMSuThirdRwStFwdBkwdPosDelta_Val
  PA_KeSMSuThrdRwCushFoldPosDelta_Val : Constant  Value=KeSMSuThrdRwCushFoldPosDelta_Val
  PA_KeSMSuThrdRwStBackPosDelta_Val : Constant  Value=KeSMSuThrdRwStBackPosDelta_Val
  PA_KeSMSwDltTrgtPos_Val10 : Constant  OutDataTypeStr=boolean
  PA_KeSMSwDltTrgtPos_Val{3,6,8,18} (4 alike) : Constant  Value=KeSMSwPosInvalidVal_Val
  PA_KeSMSwDltTrgtPos_Val2 : Constant  Value=0  OutDataTypeStr=boolean
  PA_KeSMSwDltTrgtPos_Val24 : Constant  Value=0  OutDataTypeStr=boolean
  PA_KeSMSwDltTrgtPos_Val9 : Constant  Value=SeatChldLkSt.ChldLkSt_Unlock
  R3RtReclnUpDn_Step1 : Lib/CommonUsed  SystemSampleTime=-1
  R3Rt_FrwdBkwd_Step2 : Lib/CommonUsed  SystemSampleTime=-1
  Relational Operator1 : RelationalOperator  Operator=~=  OutDataTypeStr=boolean  RndMeth=Simplest
  Relational Operator5 : RelationalOperator  Operator=~=  OutDataTypeStr=boolean  RndMeth=Simplest
  Switch1 : Switch  Criteria=u2 ~= 0
  Unit Delay : UnitDelay  SampleTime=-1
  R3Rt_Step1_ini : Outport
  R3Rt__Step1done : Outport  Port=2
  IfVeSMSbThdRwRtStRclCmdSrv_Val_writeRaw : Outport  Port=3
  R3Rt_TrgtPoss : Outport  Port=4  VectorParamsAs1DForOutWhenUnconnected=on
  R3Rt_All_done : Outport  Port=5
  R3Rt_SpdCtrl : Outport  Port=6  VectorParamsAs1DForOutWhenUnconnected=on
  wires:
  PA_KeSMSwDltTrgtPos_Val2/1 -> R3RtReclnUpDn_Step1/13
  PA_KeSMSwDltTrgtPos_Val24/1 -> R3Rt_FrwdBkwd_Step2/13
  Bus Selector2/8 -> [K_FrwdBkwdPosMax]  "<FrwdBkwdPosMax>"
  Bus Selector2/1 -> [K_BkReclnUpwdDnwdPos]  "<BkReclnUpwdDnwdPos>"
  Bus Selector2/2 -> [K_BkReclnUpwdDnwdPosMax]  "<BkReclnUpwdDnwdPosMax>"
  Bus Selector2/9 -> [K_FrwdBkwdPosMin]  "<FrwdBkwdPosMin>"
  Bus Selector3/1 -> Bus Selector2/1  "<VIPThdRwRtSt>"
  Bus Selector2/3 -> [K_BkReclnUpwdDnwdPosMin]  "<BkReclnUpwdDnwdPosMin>"
  ModeStCalib_3R/1 -> Bus Selector3/1
  Bus Selector2/5 -> [K_CshnFldUpwdDnwdPosMax]  "<CshnFldUpwdDnwdPosMax>"
  Bus Selector2/7 -> [K_FrwdBkwdPos]  "<FrwdBkwdPos>"
  Bus Selector2/4 -> [K_CshnFldUpwdDnwdPos]  "<CshnFldUpwdDnwdPos>"
  Bus Selector2/6 -> [K_CshnFldUpwdDnwdPosMin]  "<CshnFldUpwdDnwdPosMin>"
  [KeSMSuMdMotFinshdTm_Val] -> R3Rt_FrwdBkwd_Step2/12
  [KeSMSuMdMotFinshdTm_Val] -> R3RtReclnUpDn_Step1/12
  PA_KeSMSuModeReqDurgTm_Val/1 -> [Tick]
  PA_KeSMSuMdMotFinshdTm_Val/1 -> [KeSMSuMdMotFinshdTm_Val]
  PA_KeSMSuThrdRwStBackPosDelta_Val/1 -> [KeSMSuThrdRwStBackPosDelta_Val]
  PA_KeSMSuThirdRwStFwdBkwdPosDelta_Val/1 -> [KeSMSuThirdRwStFwdBkwdPosDelta_Val]
  PA_KeSMSuThrdRwCushFoldPosDelta_Val/1 -> [KeSMSuThrdRwCushFoldPosDelta_Val]
  [R3Rt__Step1done] -> R3Rt_All_done/1
  Logical Operator6/1 -> [R3Rt__Step1done], R3Rt__Step1done/1
  Unit Delay/1 -> Logical Operator6/2
  [Step1En] -> R3Rt_FrwdBkwd_Step2/2
  Logical Operator4/1 -> Unit Delay/1
  [Step1_2_done] -> Logical Operator4/2
  [Step1_1_done] -> Logical Operator4/1
  [R3Rt_Step1_2_ini] -> Logical Operator/2
  Logical Operator/1 -> R3Rt_Step1_ini/1, Logical Operator6/1
  [R3Rt_Step1_1_ini] -> Logical Operator/1
  R3RtReclnUpDn_Step1/1 -> [R3Rt_Step1_1_ini]
  [K_BkReclnUpwdDnwdPosMax] -> R3RtReclnUpDn_Step1/5
  [Trig] -> R3RtReclnUpDn_Step1/1
  Mode_Trig/1 -> [Trig]
  [KeSMSuThrdRwStBackPosDelta_Val] -> R3RtReclnUpDn_Step1/7
  [ThdRwRtStFrwdBkwdPos] -> R3Rt_FrwdBkwd_Step2/3
  [K_FrwdBkwdPosMax] -> R3Rt_FrwdBkwd_Step2/5
  [KeSMSuThirdRwStFwdBkwdPosDelta_Val] -> R3Rt_FrwdBkwd_Step2/7
  [K_FrwdBkwdPosMin] -> R3Rt_FrwdBkwd_Step2/4
  R3Rt_FrwdBkwd_Step2/1 -> [R3Rt_Step1_2_ini]
  R3Rt_FrwdBkwd_Step2/2 -> [Step2ArrivedTarPos]
  [K_BkReclnUpwdDnwdPosMin] -> R3RtReclnUpDn_Step1/4
  R3RtReclnUpDn_Step1/2 -> [Step1ArrivedTarPos]
  [ThdRwRtStBkReclnUpwdDnwdPos] -> R3RtReclnUpDn_Step1/3
  [K_BkReclnUpwdDnwdPos] -> R3RtReclnUpDn_Step1/6
  [ThdRwRtStBkReclnUpwdDnwdPosV] -> R3RtReclnUpDn_Step1/8
  PA_KeSMSwDltTrgtPos_Val3/1 -> R3RtReclnUpDn_Step1/10
  R3RtReclnUpDn_Step1/3 -> [R3RtReclnUpDn_TarPos]
  R3RtReclnUpDn_Step1/4 -> [Step1_1_done]
  Step1En/1 -> [Step1En], R3RtReclnUpDn_Step1/2
  [Trig] -> R3Rt_FrwdBkwd_Step2/1
  [K_FrwdBkwdPos] -> R3Rt_FrwdBkwd_Step2/6
  [ThdRwRtStFrwdBkwdPosV] -> R3Rt_FrwdBkwd_Step2/8
  [isSeatOccupied] -> R3RtReclnUpDn_Step1/9
  [isSeatOccupied] -> R3Rt_FrwdBkwd_Step2/9
  PA_KeSMSwDltTrgtPos_Val6/1 -> R3Rt_FrwdBkwd_Step2/10
  [Tick] -> R3RtReclnUpDn_Step1/11
  [Tick] -> R3Rt_FrwdBkwd_Step2/11
  R3Rt_FrwdBkwd_Step2/3 -> [R3Rt_FrwdBkwd_TarPos]
  R3Rt_FrwdBkwd_Step2/4 -> [Step1_2_done]
  PA_KeSMSwDltTrgtPos_Val10/1 -> IfVeSMSbThdRwRtStRclCmdSrv_Val_writeRaw/1
  Bus Selector1/1 -> [ThdRwRtStBkReclnUpwdDnwdPosV]  "<IfVeSMSuThdRwRtStBkReclnUpwdDnwdPosV_Val_read>"
  Bus Selector/3 -> [ThdRwRtStFrwdBkwdPos]  "<IfVeSMSuThdRwRtStFrwdBkwdPos_Val_read>"
  ThdRwRtStPossV/1 -> Bus Selector1/1
  ThdRwRtStPoss/1 -> Bus Selector/1
  Bus Selector/2 -> [ThdRwRtStCshnFldUpwdDnwdPos]  "<IfVeSMSuThdRwRtStCshnFldUpwdDnwdPos_Val_read>"
  Bus Selector/1 -> [ThdRwRtStBkReclnUpwdDnwdPos]  "<IfVeSMSuThdRwRtStBkReclnUpwdDnwdPos_Val_read>"
  Bus Selector1/2 -> [ThdRwRtStCshnFldUpwdDnwdPosV]  "<IfVeSMSuThdRwRtStCshnFldUpwdDnwdPosV_Val_read>"
  Bus Selector1/3 -> [ThdRwRtStFrwdBkwdPosV]  "<IfVeSMSuThdRwRtStFrwdBkwdPosV_Val_read>"
  PA_KeSMSwDltTrgtPos_Val8/1 -> Bus Creator/2  "ThdRwRtStCshnFldUpwdDnwdTrgtPos"
  [R3RtReclnUpDn_TarPos] -> Bus Creator/1  "ThdRwRtStBkReclnUpwdDnwdTrgtPos"
  [R3Rt_FrwdBkwd_TarPos] -> Bus Creator/3  "ThdRwRtStFrwdBkwdTrgtPos"
  Bus Creator/1 -> R3Rt_TrgtPoss/1
  Bus Selector4/1 -> [BkReclnUpwdDnwdMovConfig]  "<BkReclnUpwdDnwdMovConfig>"
  StConfig/1 -> Bus Selector4/1
  Bus Selector4/2 -> [CshnFldUpwdDnwdMovConfig]  "<CshnFldUpwdDnwdMovConfig>"
  Bus Selector4/3 -> [FrwdBkwdMovConfig]  "<FrwdBkwdMovConfig>"
  [FrwdBkwdMovConfig] -> R3Rt_FrwdBkwd_Step2/14
  [BkReclnUpwdDnwdMovConfig] -> R3RtReclnUpDn_Step1/14
  PA_KeSMSwDltTrgtPos_Val9/1 -> Relational Operator1/2
  SecRwRtStChldLkRsp_L/1 -> Relational Operator1/1
  Logical Operator9/1 -> [isSeatOccupied]
  Relational Operator1/1 -> Logical Operator9/2
  SeatOccupied/1 -> Logical Operator9/1
  [CntLow] -> R3RtReclnUpDn_Step1/15
  [CntLow] -> R3Rt_FrwdBkwd_Step2/15
  PA_KeSMSuMdRetryTm1_Val/1 -> [CntLow]
  Switch1/1 -> R3Rt_SpdCtrl/1
  Relational Operator5/1 -> Switch1/2
  Constant/1 -> Switch1/1
  Constant1/1 -> Switch1/3
  [R3Rt_FrwdBkwd_TarPos] -> Relational Operator5/1  "ThdRwLtStFrwdBkwdTrgtPos"
  PA_KeSMSwDltTrgtPos_Val18/1 -> Relational Operator5/2
